simulink model "dataRecorder"  (R2024b)
settings: Solver=VariableStepAuto  StartTime=0.0  StopTime=inf  RelTol=1e-3
InitFcn:
  | my_callback
libraries: etargetslib x1, sldrtlib x1, dspnetwork x1
settings Model: Creator=pablo  LastModifiedBy=AERO-REMOTELABS
settings SolverCC: AlgebraicLoopSolver=TrustRegion
settings DebuggingCC: UnconnectedInputMsg=warning  UnconnectedOutputMsg=warning  UnconnectedLineMsg=warning
settings ModelReferenceCC: EnableRefExpFcnMdlSchedulingChecks=on
settings RTWCC: GPUComputeCapability=3.5  DLArmComputeVersion=19.05

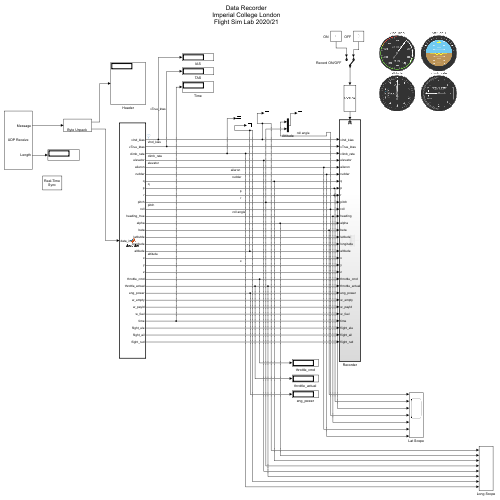
[thumbnail: Simulink's stored preview of the top-level diagram]
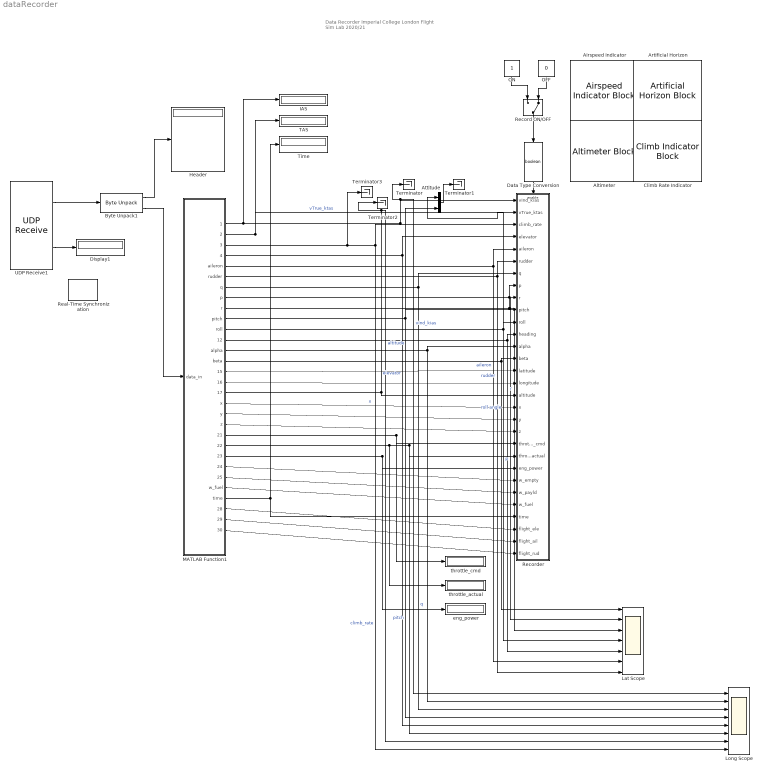
== system dataRecorder ==
  note: Data Recorder
      | Imperial College London
      | Flight Sim Lab 2020/21
  Airspeed Indicator : AirspeedIndicatorBlock  ScaleMin=0  ScaleMax=450
  Altimeter : AltimeterBlock
  Artificial Horizon : ArtificialHorizonBlock
  Attitude : Mux  Inputs=2
  Byte Unpack1 : etargetslib/Byte Unpack  dimensions={5,[9,15]}  datatypes={'uint8','single'}  byteAlign=1
  Climb Rate Indicator : ClimbIndicatorBlock
  Data Type Conversion : DataTypeConversion  OutDataTypeStr=boolean  SaturateOnIntegerOverflow=off  RndMeth=Floor
  Display1 : Display
  Header : Display
  IAS : Display
  Lat Scope : Scope  NumInputPorts=7
  Long Scope : Scope  NumInputPorts=8
  MATLAB Function1 : MATLAB Function  TreatAsAtomicUnit=on
  OFF : Constant  Value=0
  ON : Constant
  Real-Time Synchronization : sldrtlib/Real-Time Synchronization  SampleTime=0.0125  MaxMissedTicks=1000  ShowMissedTicks=off  YieldWhenWaiting=off
  Record ON/OFF : ManualSwitch  CurrentSetting=0
  Recorder : Subsystem
  TAS : Display
  Terminator{,1..3} (4 alike) : Terminator
  Time : Display
  UDP Receive1 : dspnetwork/UDP Receive  localURL='0.0.0.0'  localPort=49300  remoteURL='192.168.5.221'  remotePort=-1  recvBufferSize=8192  dims=545  signalDatatype=uint8  isComplex=off  isVarSize=off  showBlockingTime=off  blockingTime=0  sampletime=0.0125  blockPlatform=[]
  eng_power : Display
  throttle_actual : Display
  throttle_cmd : Display
  wires:
  MATLAB Function1/30(flight_rud) -> Recorder/30(flight_rud)
  MATLAB Function1/20(z) -> Recorder/20(z)
  OFF/1 -> Record ON/OFF/2
  MATLAB Function1/27(time) -> Time/1, Recorder/27(time)
  MATLAB Function1/29(flight_ail) -> Recorder/29(flight_ail)
  ON/1 -> Record ON/OFF/1
  Byte Unpack1/1 -> Header/1
  MATLAB Function1/28(flight_ele) -> Recorder/28(flight_ele)
  MATLAB Function1/16(longitude) -> Recorder/16(longitude)
  MATLAB Function1/4(elevator) -> Recorder/4(elevator), Long Scope/5  "elevator"
  Record ON/OFF/1 -> Data Type Conversion/1
  Data Type Conversion/1 -> Recorder/Enable
  MATLAB Function1/24(w_empty) -> Recorder/24(w_empty)
  MATLAB Function1/19(y) -> Recorder/19(y)
  Byte Unpack1/2 -> MATLAB Function1/1(data_in)
  MATLAB Function1/10(pitch) -> Attitude/2, Long Scope/4, Recorder/10(pitch)  "pitch"
  MATLAB Function1/9(r) -> Lat Scope/3, Recorder/9(r)  "r"
  MATLAB Function1/26(w_fuel) -> Recorder/26(w_fuel)
  UDP Receive1/1 -> Byte Unpack1/1
  UDP Receive1/2 -> Display1/1
  MATLAB Function1/17(altitude) -> Terminator2/1, Long Scope/7, Recorder/17(altitude)  "altitude"
  MATLAB Function1/11(roll) -> Attitude/1, Recorder/11(roll), Lat Scope/4  "roll angle"
  MATLAB Function1/14(beta) -> Recorder/14(beta), Lat Scope/1
  MATLAB Function1/6(rudder) -> Recorder/6(rudder), Lat Scope/7  "rudder"
  MATLAB Function1/15(latitutde) -> Recorder/15(latitude)
  MATLAB Function1/3(climb_rate) -> Recorder/3(climb_rate), Long Scope/8, Terminator3/1  "climb_rate"
  MATLAB Function1/12(heading_true) -> Recorder/12(heading), Lat Scope/5
  MATLAB Function1/23(eng_power) -> eng_power/1, Recorder/23(eng_power)
  MATLAB Function1/22(throttle_actual) -> throttle_actual/1, Long Scope/6, Recorder/22(throttle_actual)
  MATLAB Function1/8(p) -> Recorder/8(p), Lat Scope/2  "p"
  MATLAB Function1/18(x) -> Recorder/18(x)  "x"
  MATLAB Function1/7(q) -> Long Scope/3, Recorder/7(q)  "q"
  MATLAB Function1/5(aileron) -> Recorder/5(aileron), Lat Scope/6  "aileron"
  MATLAB Function1/25(w_payld) -> Recorder/25(w_payld)
  MATLAB Function1/13(alpha) -> Long Scope/2, Recorder/13(alpha)
  MATLAB Function1/1(vInd_kias) -> IAS/1, Recorder/1(vInd_kias), Terminator/1, Long Scope/1  "vInd_kias"
  MATLAB Function1/2(vTrue_ktas) -> TAS/1, Recorder/2(vTrue_ktas)  "vTrue_ktas"
  MATLAB Function1/21(throttle_cmd) -> throttle_cmd/1, Recorder/21(throttle_cmd)
  Attitude/1 -> Terminator1/1

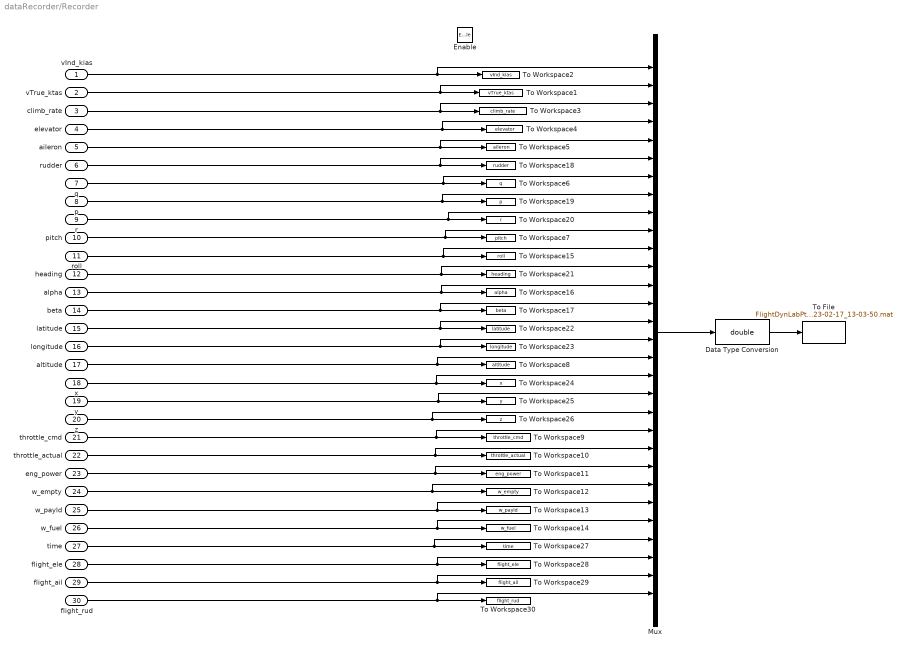
== system dataRecorder/Recorder ==
  vInd_kias : Inport
  vTrue_ktas : Inport  Port=2
  climb_rate : Inport  Port=3
  elevator : Inport  Port=4
  aileron : Inport  Port=5
  rudder : Inport  Port=6
  q : Inport  Port=7
  p : Inport  Port=8
  r : Inport  Port=9
  pitch : Inport  Port=10
  roll : Inport  Port=11
  heading : Inport  Port=12
  alpha : Inport  Port=13
  beta : Inport  Port=14
  latitude : Inport  Port=15
  longitude : Inport  Port=16
  altitude : Inport  Port=17
  x : Inport  Port=18
  y : Inport  Port=19
  z : Inport  Port=20
  throttle_cmd : Inport  Port=21
  throttle_actual : Inport  Port=22
  eng_power : Inport  Port=23
  w_empty : Inport  Port=24
  w_payld : Inport  Port=25
  w_fuel : Inport  Port=26
  time : Inport  Port=27
  flight_ele : Inport  Port=28
  flight_ail : Inport  Port=29
  flight_rud : Inport  Port=30
  Enable : EnablePort
  Data Type Conversion : DataTypeConversion  OutDataTypeStr=double  SaturateOnIntegerOverflow=off  RndMeth=Floor
  Mux : Mux  Inputs=30
  To File : ToFile  Filename=FlightDynLabPt1_2023-02-17_13-03-50.mat  MatrixName=data  SaveFormat=Timeseries
  To Workspace1 : ToWorkspace  VariableName=vTrue_ktas  SampleTime=-1
  To Workspace10 : ToWorkspace  VariableName=throttle_actual  SampleTime=-1
  To Workspace11 : ToWorkspace  VariableName=eng_power  SampleTime=-1
  To Workspace12 : ToWorkspace  VariableName=w_empty  SampleTime=-1
  To Workspace13 : ToWorkspace  VariableName=w_payld  SampleTime=-1
  To Workspace14 : ToWorkspace  VariableName=w_fuel  SampleTime=-1
  To Workspace15 : ToWorkspace  VariableName=roll  SampleTime=-1
  To Workspace16 : ToWorkspace  VariableName=alpha  SampleTime=-1
  To Workspace17 : ToWorkspace  VariableName=beta  SampleTime=-1
  To Workspace18 : ToWorkspace  VariableName=rudder  SampleTime=-1
  To Workspace19 : ToWorkspace  VariableName=p  SampleTime=-1
  To Workspace2 : ToWorkspace  VariableName=vInd_kias  SampleTime=-1
  To Workspace20 : ToWorkspace  VariableName=r  SampleTime=-1
  To Workspace21 : ToWorkspace  VariableName=heading  SampleTime=-1
  To Workspace22 : ToWorkspace  VariableName=latitude  SampleTime=-1
  To Workspace23 : ToWorkspace  VariableName=longitude  SampleTime=-1
  To Workspace24 : ToWorkspace  VariableName=x  SampleTime=-1
  To Workspace25 : ToWorkspace  VariableName=y  SampleTime=-1
  To Workspace26 : ToWorkspace  VariableName=z  SampleTime=-1
  To Workspace27 : ToWorkspace  VariableName=time  SampleTime=-1
  To Workspace28 : ToWorkspace  VariableName=flight_ele  SampleTime=-1
  To Workspace29 : ToWorkspace  VariableName=flight_ail  SampleTime=-1
  To Workspace3 : ToWorkspace  VariableName=climb_rate  SampleTime=-1
  To Workspace30 : ToWorkspace  VariableName=flight_rud  SampleTime=-1
  To Workspace4 : ToWorkspace  VariableName=elevator  SampleTime=-1
  To Workspace5 : ToWorkspace  VariableName=aileron  SampleTime=-1
  To Workspace6 : ToWorkspace  VariableName=q  SampleTime=-1
  To Workspace7 : ToWorkspace  VariableName=pitch  SampleTime=-1
  To Workspace8 : ToWorkspace  VariableName=altitude  SampleTime=-1
  To Workspace9 : ToWorkspace  VariableName=throttle_cmd  SampleTime=-1
  wires:
  pitch/1 -> Mux/10, To Workspace7/1
  z/1 -> Mux/20, To Workspace26/1
  q/1 -> Mux/7, To Workspace6/1
  vInd_kias/1 -> Mux/1, To Workspace2/1
  beta/1 -> Mux/14, To Workspace17/1
  longitude/1 -> Mux/16, To Workspace23/1
  climb_rate/1 -> Mux/3, To Workspace3/1
  vTrue_ktas/1 -> Mux/2, To Workspace1/1
  heading/1 -> Mux/12, To Workspace21/1
  w_fuel/1 -> Mux/26, To Workspace14/1
  r/1 -> Mux/9, To Workspace20/1
  w_payld/1 -> Mux/25, To Workspace13/1
  altitude/1 -> Mux/17, To Workspace8/1
  aileron/1 -> Mux/5, To Workspace5/1
  w_empty/1 -> Mux/24, To Workspace12/1
  alpha/1 -> Mux/13, To Workspace16/1
  p/1 -> Mux/8, To Workspace19/1
  throttle_cmd/1 -> Mux/21, To Workspace9/1
  rudder/1 -> Mux/6, To Workspace18/1
  eng_power/1 -> Mux/23, To Workspace11/1
  elevator/1 -> Mux/4, To Workspace4/1
  roll/1 -> Mux/11, To Workspace15/1
  throttle_actual/1 -> Mux/22, To Workspace10/1
  y/1 -> Mux/19, To Workspace25/1
  latitude/1 -> Mux/15, To Workspace22/1
  x/1 -> Mux/18, To Workspace24/1
  time/1 -> Mux/27, To Workspace27/1
  flight_ele/1 -> Mux/28, To Workspace28/1
  flight_ail/1 -> Mux/29, To Workspace29/1
  flight_rud/1 -> Mux/30, To Workspace30/1
  Mux/1 -> Data Type Conversion/1
  Data Type Conversion/1 -> To File/1

== matlab function dataRecorder/MATLAB Function1 ==
  data: vInd_kias output; vTrue_ktas output; climb_rate output; elevator output; aileron output; rudder output; q output; p output; r output; pitch output; roll output; heading_true output; alpha output; beta output; latitutde output; longitude output; altitude output; x output; y output; z output; throttle_cmd output; throttle_actual output; eng_power output; w_empty output; w_payld output; w_fuel output; time output; data_in input; flight_ele output; flight_ail output; flight_rud output
function [vInd_kias,vTrue_ktas,...
    climb_rate,...
    elevator,aileron,rudder,...
    q,p,r,...
    pitch, roll, heading_true,...
    alpha,beta,...
    latitutde, longitude, altitude,...
    x,y,z,...
    throttle_cmd,...
    throttle_actual,...
    eng_power,...
    w_empty,w_payld,w_fuel,...
    time,...
    flight_ele,flight_ail,flight_rud] = decoder(data_in)
 frame_rate = data_in(2,1);
 time = data_in(2,2);
 vInd_kias = data_in(2,3);
 vTrue_ktas = data_in(4,3);
 climb_rate = data_in(4,4);
 elevator = data_in(2,5); %Joystick elevator value
 aileron = data_in(3,5);  %Joystick aileron value
 rudder= data_in(4,5);    %Joystick rudder value
 flight_ele = data_in(2,6);
 flight_ail = data_in(3,6);
 flight_rud = data_in(4,6);
 q= data_in(2,7);
 p= data_in(3,7);
 r= data_in(4,7);
 pitch= data_in(2,8);
 roll= data_in(3,8);
 heading_true= data_in(4,8);
 alpha = data_in(2,9);
 beta  = data_in(3,9);
 latitutde= data_in(2,10);
 longitude= data_in(3,10);
 altitude= data_in(4,10);
 x = data_in(2,11);
 y = data_in(3,11);
 z = data_in(4,11);
 throttle_cmd = data_in(2,12);
 throttle_actual = data_in(2,13);
 eng_power = data_in(2,14);
 w_empty = data_in(2,15);
 w_payld = data_in(3,15);
 w_fuel  = data_in(4,15);
end
